simulink model "IndustrialMicrogrid"  (R2023a)
settings: Solver=FixedStepDiscrete  StartTime=0.0  StopTime=10  FixedStep=Ts  RelTol=1e-3
PostLoadFcn:
  | IndustrialMicrogridInputData
  | GfmGridFormingConverterInputParameters
model workspace (MAT data in the model file):
  caseNum = 2
undefined symbols (not defined in the file): base, BESS, DiscIntNeverNeededParam, grid, Grid, gridInverter, machine, microgrid, PV, PVInverter, PVTransformer, scrFactorRg, scrFactorXg, transformer, Ts
libraries: ee_lib x112, eeGeneralControl x104, nesl_utility_internal x64, simulink x56, nesl_utility x37, fl_lib x29, slpidlib x13, eeTransforms x11, eeTotalHarmonicDistorsion x8, eeRmsMeasurement x4, eeSinusoidalMeasurement x4, simulink_extras x2
(part 6 of 14)

== system IndustrialMicrogrid/MG2 Primary Substation/Microgrid Controller 2/Breaker Control  ==
  Bus Element In1 : Inport  PortName=Control Room  Element=ResynchCmd2
  Bus Element In3 : Inport  PortName=Control Room  Element=PlannedIslandCmd2
  Bus Element In6 : Inport  PortName=Control Room  Element=BRKcontrol2
  Bus Element In4 : Inport  PortName=Control Room  Element=BRKcontrol2
  Bus Element In5 : Inport  Port=2  PortName=MGController  Element=IslandMGController2.MGPlannedIsland2.plannedisland
  Bus Element In2 : Inport  Port=2  PortName=MGController  Element=ResynchMGController2.MGResynch2.resynch
  Cast To Double1 : DataTypeConversion  OutDataTypeStr=double  SaturateOnIntegerOverflow=off  RndMeth=Floor
  Logical Operator1 : Logic  Operator=NOT  AllPortsSameDT=off  OutDataTypeStr=boolean
  Logical Operator{2..5} (4 alike) : Logic  AllPortsSameDT=off  OutDataTypeStr=boolean
  Logical Operator6 : Logic  Operator=OR  AllPortsSameDT=off  OutDataTypeStr=boolean
  Logical Operator7 : Logic  Operator=NOT  AllPortsSameDT=off  OutDataTypeStr=boolean
  Breaker : Outport
  wires:
  Logical Operator7/1 -> Logical Operator5/1
  Logical Operator1/1 -> Logical Operator4/1
  Logical Operator5/1 -> Logical Operator6/2
  Logical Operator4/1 -> Logical Operator6/1
  Bus Element In6/1 -> Logical Operator1/1
  Logical Operator6/1 -> Cast To Double1/1
  Bus Element In4/1 -> Logical Operator5/2
  Logical Operator2/1 -> Logical Operator7/1
  Logical Operator3/1 -> Logical Operator4/2
  Bus Element In5/1 -> Logical Operator3/2
  Bus Element In3/1 -> Logical Operator3/1
  Bus Element In1/1 -> Logical Operator2/1
  Bus Element In2/1 -> Logical Operator2/2
  Cast To Double1/1 -> Breaker/1

== system IndustrialMicrogrid/MG2 Primary Substation/Microgrid Controller 2/Frequency Reference ==
  Bus Element In : Inport  PortName=Control Room  Element=ResynchCmd2
  Bus Element In1 : Inport  PortName=Control Room  Element=PowerCmd2
  Bus Element In4 : Inport  PortName=Control Room  Element=BlackStartMG2
  Bus Element In3 : Inport  Port=2  PortName=MGController  Element=BlackStart.Fref2
  Bus Element In2 : Inport  Port=2  PortName=MGController  Element=ResynchMGController2.MGResynch2.synchfrequency
  Constant : Constant  Value=IslandFrequency
  Constant1 : Constant  Value=GridFrequency
  Gain1 : Gain  Gain=1/60
  Sum : Sum  Inputs=|++
  Switch : Switch  Criteria=u2 > Threshold  Threshold=0.5  SaturateOnIntegerOverflow=off  InputSameDT=off
  Switch1 : Switch  Criteria=u2 > Threshold  Threshold=0.5  SaturateOnIntegerOverflow=off  InputSameDT=off
  Switch2 : Switch  Criteria=u2 > Threshold  Threshold=0.5  SaturateOnIntegerOverflow=off  InputSameDT=off
  fref : Outport
  wires:
  Bus Element In4/1 -> Switch1/2
  Constant1/1 -> Switch2/1
  Switch1/1 -> Gain1/1
  Constant/1 -> Sum/2, Switch/3
  Gain1/1 -> fref/1
  Bus Element In2/1 -> Sum/1
  Bus Element In/1 -> Switch/2
  Bus Element In1/1 -> Switch2/2
  Bus Element In3/1 -> Switch1/1
  Switch2/1 -> Switch1/3
  Sum/1 -> Switch/1
  Switch/1 -> Switch2/3

== system IndustrialMicrogrid/MG2 Primary Substation/Microgrid Controller 2/PLL  ==
  In Bus Element : Inport  PortName=mPCC2  Element=Gridvoltage
  In Bus Element1 : Inport  PortName=mPCC2  Element=mPCC2.voltage
  PLL : Subsystem
  PLL start at 0.2 s : Subsystem
  PLL starts at 0.2 s : Subsystem
  PLL1 : Subsystem
  Bus Element Out : Outport  PortName=Grid2  Element=frequency
  Bus Element Out1 : Outport  PortName=Grid2  Element=angle
  Bus Element Out2 : Outport  PortName=Grid2  Element=voltage
  Bus Element Out3 : Outport  Port=2  PortName=Island2  Element=voltage
  Bus Element Out4 : Outport  Port=2  PortName=Island2  Element=frequency
  Bus Element Out5 : Outport  Port=2  PortName=Island2  Element=angle
  wires:
  PLL1/3(mag) -> Bus Element Out3/1
  PLL1/2(angle) -> Bus Element Out5/1
  PLL1/1(fre) -> Bus Element Out4/1
  PLL/3(mag) -> Bus Element Out2/1
  PLL/2(angle) -> Bus Element Out1/1
  PLL/1(fre) -> Bus Element Out/1
  PLL start at 0.2 s/1(Out1) -> PLL/1(abc)
  In Bus Element1/1 -> PLL starts at 0.2 s/1(PCC measurement)
  PLL starts at 0.2 s/1(abc) -> PLL1/1(abc)
  In Bus Element/1 -> PLL start at 0.2 s/1(PCC measurement)

== system IndustrialMicrogrid/MG2 Primary Substation/Microgrid Controller 2/Planned Island ==
  Control Room : Inport
  mPCCPLL 2 : Inport  Port=2
  Bus Creator : BusCreator  Inputs=2
  Control for Zero Powerflow1 : Subsystem  mask(Planned island control parameters){KpPPlannedIsland=microgrid.KpPPlannedIsland2, KiPPlannedIsland=microgrid.KiPPlannedIsland2, KpQPlannedIsland=microgrid.KpQPlannedIsland2, KiQPlannedIsland=microgrid.KiQPlannedIsland2, ZeroActivePowerThreshold=microgrid.zeroActivePowerThreshold2, ZeroReactivePowerThreshold=microgrid.zeroReactivePowerThreshold2, PlannedIslandDelay=microgrid.plannedIslandDelay}
      mask prompts: KpPPlannedIsland "Active Power Planned Island Proportional Gain"; KiPPlannedIsland "Active Power Planned Island Integral Gain"; KpQPlannedIsland "Reactive Power Planned Island Proportional Gain"; KiQPlannedIsland "Reactive Power Planned Island Intergal Gain"; ZeroActivePowerThreshold "Zero Active Power Threshold"; ZeroReactivePowerThreshold "Zero Reactive Power Threshold"; PlannedIslandDelay "Planned Island Delay"
      mask help: Provide planned island control parameters
  IslandMGController2 : Outport
  wires:
  mPCCPLL 2/1 -> Control for Zero Powerflow1/2(mPCCPLL2), Bus Creator/2  "PCC measurments2"
  Control for Zero Powerflow1/1(MGController2) -> Bus Creator/1  "MGPlannedIsland2"
  Bus Creator/1 -> IslandMGController2/1  "IslandMGController2"
  Control Room/1 -> Control for Zero Powerflow1/1(ControlRoom)

== system IndustrialMicrogrid/MG2 Primary Substation/Microgrid Controller 2/Resynchronization ==
  Control Room : Inport
  mPCCPLL : Inport  Port=2
  BESS : Inport  Port=3
  Bus Creator : BusCreator  Inputs=2
  Frequency and voltage matching : Subsystem  mask(Resynchronization control parameters){GridFrequency=grid.frequency, RadToDegree=microgrid.radToDegree, KpFreResynch=microgrid.KpFreResynch2, KiFreResynch=microgrid.KiFreResynch2, KpVolResynch=microgrid.KpVolResynch2, KiVolResynch=microgrid.KiVolResynch2, KpAngResynch=microgrid.KpAngResynch2, KiAngResynch=microgrid.KiAngResynch2, FrequencyThreshold=microgrid.frequencyThreshold, AngleThreshold=microgrid.angleThreshold, VoltageThreshold=microgrid.voltageThreshold, ResynchDelay=microgrid.resynchDelay, kDroop=microgrid.KDroop}
      mask prompts: GridFrequency "Grid Frequency"; RadToDegree "Rad to Degree"; KpFreResynch "Frequency Resynch Proportional Gain"; KiFreResynch "Frequency Resynch Integral Gain"; KpVolResynch "Voltage Resynch Proportional Gain"; KiVolResynch "Voltage Resynch Integral Gain"; KpAngResynch "Angle Resynch Proportional Gain"; KiAngResynch "Angle Resynch Integral Gain"; FrequencyThreshold "Frequency Matching Threshold"; AngleThreshold "Angle Matching Threshold"; VoltageThreshold "Voltage Matching Threshold"; ResynchDelay "Resynch Delay"; kDroop "Voltage Droop"
      mask help: Provide resynchronization control parameters
  ResynchMGController2 : Outport
  wires:
  Control Room/1 -> Frequency and voltage matching/2(ControlRoom)
  Bus Creator/1 -> ResynchMGController2/1  "ResynchMGController2"
  Frequency and voltage matching/1(MGController2) -> Bus Creator/1  "MGResynch2"
  BESS/1 -> Frequency and voltage matching/1(BESS2)
  mPCCPLL/1 -> Bus Creator/2, Frequency and voltage matching/3(mPCCPLL2)  "PCC measurments2"

== system IndustrialMicrogrid/MG2 Primary Substation/Microgrid Controller 2/Voltage Reference ==
  Bus Element In1 : Inport  PortName=Control Room  Element=ResynchCmd2
  Bus Element In2 : Inport  PortName=Control Room  Element=BlackStartMG2
  Bus Element In4 : Inport  Port=2  PortName=MGController  Element=BlackStart.Vref2
  Bus Element In3 : Inport  Port=2  PortName=MGController  Element=ResynchMGController2.MGResynch2.synchvoltagedpr
  Constant9 : Constant  Value=IslandVoltage
  Switch1 : Switch  Criteria=u2 > Threshold  Threshold=0.5  SaturateOnIntegerOverflow=off  InputSameDT=off
  Switch2 : Switch  Criteria=u2 > Threshold  Threshold=0.5  SaturateOnIntegerOverflow=off  InputSameDT=off
  Vref : Outport
  wires:
  Bus Element In3/1 -> Switch1/1
  Constant9/1 -> Switch1/3
  Switch2/1 -> Vref/1
  Bus Element In2/1 -> Switch2/2
  Bus Element In1/1 -> Switch1/2
  Bus Element In4/1 -> Switch2/1
  Switch1/1 -> Switch2/3

== system IndustrialMicrogrid/MG2 Primary Substation/PCC Measurements and PCC Breaker/Grid Current Measurement ==
  Current and Voltage Sensor (Three-Phase)1 : ee_lib/Sensors & Transducers/Current and Voltage Sensor (Three-Phase)  vMeasurementType=ee.enum.vmeasurement.ll  outputUnit=ee.enum.unit.pu  SRated=2.5e6 A*V  VRated=microgrid.voltage V  I_specify=off  I_priority=None  I=[0, 0, 0] A  I_nominal_specify=off  I_nominal_unit=A  I_nominal_value=1  V_specify=off  V_priority=None  V=[0, 0, 0] V  V_nominal_specify=off  V_nominal_unit=V  V_nominal_value=1
      settings: InternalSimscapePortConfiguration="{\"Bottom\":[],\"Left\":[{\"id\":\"N1\",\"label\":\"~1\",\"type\":\"foundation.electrical.three_phase\"}],\"Right\":[{\"id\":\"V_output\",\"label\":\"V\",\"type\":\"output\"},{\"id\":\"I_output\",\"label\":\"I\",\"type\":\"output\"},{\"id\":\"N2\",\"label\":\"~2\",\"type\":\"foundation.electrical.three_phase\"}],\"Top\":[]}"
  PS-Simulink Converter2 : nesl_utility_internal/PS-Simulink Converter  PhysicalDomain=network_engine_domain  SubClassName=ps_output  LeftPortType=input  RightPortType=output  PseudoPeriodic=off  Frequencies=[]  VectorFormat=1-D array  Unit=V  AffineConversion=off
  PS-Simulink Converter3 : nesl_utility_internal/PS-Simulink Converter  PhysicalDomain=network_engine_domain  SubClassName=ps_output  LeftPortType=input  RightPortType=output  PseudoPeriodic=off  Frequencies=[]  VectorFormat=1-D array  Unit=A  AffineConversion=off
  Terminator : Terminator
  ~ : PMIOPort  Side=Left
  "~ " : PMIOPort  Port=2  Side=Right
  "Grid voltage 2 " : Outport
  wires:
  PS-Simulink Converter3/1 -> Terminator/1
  PS-Simulink Converter2/1 -> "Grid voltage 2 "/1
  connections:
  Current and Voltage Sensor (Three-Phase)1/RConn3 -- "~ "/RConn1
  Current and Voltage Sensor (Three-Phase)1/RConn2 -- PS-Simulink Converter3/LConn1
  ~/RConn1 -- Current and Voltage Sensor (Three-Phase)1/LConn1
  Current and Voltage Sensor (Three-Phase)1/RConn1 -- PS-Simulink Converter2/LConn1

== system IndustrialMicrogrid/MG2 Primary Substation/PCC Measurements and PCC Breaker/Grid Power Measurement ==
  Current and Voltage Sensor (Three-Phase) : ee_lib/Sensors & Transducers/Current and Voltage Sensor (Three-Phase)  vMeasurementType=ee.enum.vmeasurement.ll  outputUnit=ee.enum.unit.pu  SRated=2.5e6 A*V  VRated=microgrid.voltage V  I_specify=off  I_priority=None  I=[0, 0, 0] A  I_nominal_specify=off  I_nominal_unit=A  I_nominal_value=1  V_specify=off  V_priority=None  V=[0, 0, 0] V  V_nominal_specify=off  V_nominal_unit=V  V_nominal_value=1
      settings: InternalSimscapePortConfiguration="{\"Bottom\":[],\"Left\":[{\"id\":\"N1\",\"label\":\"~1\",\"type\":\"foundation.electrical.three_phase\"}],\"Right\":[{\"id\":\"V_output\",\"label\":\"V\",\"type\":\"output\"},{\"id\":\"I_output\",\"label\":\"I\",\"type\":\"output\"},{\"id\":\"N2\",\"label\":\"~2\",\"type\":\"foundation.electrical.three_phase\"}],\"Top\":[]}"
  Low-Pass Filter (Discrete or Continuous) : eeGeneralControl/Low-Pass Filter (Discrete or Continuous)  K=1  T=0.1  B=inf  A=-inf  init_option=Inherited from block input  x0=0  Ts=Ts
  Low-Pass Filter (Discrete or Continuous)1 : eeGeneralControl/Low-Pass Filter (Discrete or Continuous)  K=1  T=0.1  B=inf  A=-inf  init_option=Inherited from block input  x0=0  Ts=Ts
  PS-Simulink Converter : nesl_utility_internal/PS-Simulink Converter  PhysicalDomain=network_engine_domain  SubClassName=ps_output  LeftPortType=input  RightPortType=output  PseudoPeriodic=off  Frequencies=[]  VectorFormat=1-D array  Unit=inherit  AffineConversion=off
  PS-Simulink Converter1 : nesl_utility_internal/PS-Simulink Converter  PhysicalDomain=network_engine_domain  SubClassName=ps_output  LeftPortType=input  RightPortType=output  PseudoPeriodic=off  Frequencies=[]  VectorFormat=1-D array  Unit=inherit  AffineConversion=off
  PS-Simulink Converter8 : nesl_utility_internal/PS-Simulink Converter  PhysicalDomain=network_engine_domain  SubClassName=ps_output  LeftPortType=input  RightPortType=output  PseudoPeriodic=off  Frequencies=[]  VectorFormat=1-D array  Unit=MW  AffineConversion=off
  PS-Simulink Converter9 : nesl_utility_internal/PS-Simulink Converter  PhysicalDomain=network_engine_domain  SubClassName=ps_output  LeftPortType=input  RightPortType=output  PseudoPeriodic=off  Frequencies=[]  VectorFormat=1-D array  Unit=MV*A  AffineConversion=off
  Power Sensor (Three-Phase)2 : ee_lib/Sensors & Transducers/Power Sensor (Three-Phase)  load_type=ee.enum.passive.type_balanced.balanced  f0=60 Hz  config=ee.enum.with_neutral.no  rho=1
      settings: InternalSimscapePortConfiguration="{\"Bottom\":[],\"Left\":[{\"id\":\"N1\",\"label\":\"~1\",\"type\":\"foundation.electrical.three_phase\"}],\"Right\":[{\"id\":\"N2\",\"label\":\"~2\",\"type\":\"foundation.electrical.three_phase\"}],\"Top\":[{\"id\":\"Pm\",\"label\":\"P\",\"type\":\"output\"},{\"id\":\"Qm\",\"label\":\"Q\",\"type\":\"output\"}]}"
  ~ : PMIOPort  Side=Left
  "~ " : PMIOPort  Port=2  Side=Right
  Out Bus Element : Outport  PortName=mPCC2  Element=voltage
  Out Bus Element1 : Outport  PortName=mPCC2  Element=current
  Out Bus Element2 : Outport  PortName=mPCC2  Element=activepower
  Out Bus Element3 : Outport  PortName=mPCC2  Element=reactivepower
  wires:
  Low-Pass Filter (Discrete or Continuous)1/1 -> Out Bus Element3/1
  Low-Pass Filter (Discrete or Continuous)/1 -> Out Bus Element2/1
  PS-Simulink Converter1/1 -> Out Bus Element1/1
  PS-Simulink Converter/1 -> Out Bus Element/1
  PS-Simulink Converter9/1 -> Low-Pass Filter (Discrete or Continuous)1/1
  PS-Simulink Converter8/1 -> Low-Pass Filter (Discrete or Continuous)/1
  connections:
  ~/RConn1 -- Power Sensor (Three-Phase)2/LConn1
  PS-Simulink Converter8/LConn1 -- Power Sensor (Three-Phase)2/LConn2
  Current and Voltage Sensor (Three-Phase)/RConn3 -- "~ "/RConn1
  PS-Simulink Converter9/LConn1 -- Power Sensor (Three-Phase)2/LConn3
  Power Sensor (Three-Phase)2/RConn1 -- Current and Voltage Sensor (Three-Phase)/LConn1
  PS-Simulink Converter/LConn1 -- Current and Voltage Sensor (Three-Phase)/RConn1
  Current and Voltage Sensor (Three-Phase)/RConn2 -- PS-Simulink Converter1/LConn1

== system IndustrialMicrogrid/MG2 Processing, Lighting and Auxiliary Loads/Motor Loads/Subsystem ==
  Gain : Gain  Gain=60/(2*pi)
  Ideal Rotational Motion Sensor : fl_lib/Mechanical/Mechanical Sensors/Ideal Rotational Motion Sensor  reference=foundation.enum.MeasurementReference.difference  acceleration_port=false  velocity_port=true  position_port=false  wrap_angle=false  offset=0 rad
      settings: InternalSimscapePortConfiguration="{\"Bottom\":[],\"Left\":[{\"id\":\"R\",\"label\":\"R\",\"type\":\"foundation.mechanical.rotational.rotational\"}],\"Right\":[{\"id\":\"C\",\"label\":\"C\",\"type\":\"foundation.mechanical.rotational.rotational\"},{\"id\":\"W\",\"label\":\"W\",\"type\":\"output\"}],\"Top\":[]}"
  Machine Mechanical Power : ee_lib/Electromechanical/Mechanical/Machine Mechanical Power  power_sign=1  SRated=750000 A*V  FRated=60 Hz  nPolePairs=2  inputUnit=ee.enum.unit.si  torque_factor=2  inertia_option=2  J=10 kg*m^2  H=3.525 W*s/(A*V)  damper_option=2  D=39.0509 N*m*s/rad  pu_D=0.01  initialization_option=1  fMechanical0=30 Hz  fElectrical0=60 Hz
      settings: InternalSimscapePortConfiguration="{\"Bottom\":[],\"Left\":[{\"id\":\"Pm\",\"label\":\"Pm\",\"type\":\"input\"}],\"Right\":[{\"id\":\"R\",\"label\":\"R\",\"type\":\"foundation.mechanical.rotational.rotational\"},{\"id\":\"C\",\"label\":\"C\",\"type\":\"foundation.mechanical.rotational.rotational\"}],\"Top\":[]}"
  Mechanical Rotational Reference : fl_lib/Mechanical/Rotational Elements/Mechanical Rotational Reference
  PS-Simulink Converter : nesl_utility/PS-Simulink Converter  PhysicalDomain=network_engine_domain  SubClassName=ps_output  LeftPortType=input  RightPortType=output  PseudoPeriodic=off  Frequencies=[]  VectorFormat=inherit  Unit=inherit  AffineConversion=off
  Power : Constant  Value=300000  SampleTime=Ts
  Rotational Friction : fl_lib/Mechanical/Rotational Elements/Rotational Friction  brkwy_trq=25 N*m  brkwy_vel=0.1 rad/s  Col_trq=20 N*m  visc_coef=0.001 N*m*s/rad  w_specify=off  w_priority=None  w=0 rad/s  w_nominal_specify=off  w_nominal_unit=rad/s  w_nominal_value=1  t_specify=off  t_priority=None  t=0 N*m  t_nominal_specify=off  t_nominal_unit=N*m  t_nominal_value=1
  Scope : Scope
  Simulink-PS Converter2 : nesl_utility/Simulink-PS Converter  PhysicalDomain=network_engine_domain  SubClassName=ps_input  LeftPortType=input  RightPortType=output  PseudoPeriodic=off  Frequencies=[]  NoiseDistribution=none  NoiseParameters=[]  Unit=1  AffineConversion=off  FilteringAndDerivatives=provide  SimscapeFilterOrder=1  InputFilterTimeConstant=0.001  UdotUserProvided=0
  Conn1 : PMIOPort  Side=Left
  Conn2 : PMIOPort  Port=2  Side=Left
  wires:
  Power/1 -> Simulink-PS Converter2/1
  Gain/1 -> Scope/1
  PS-Simulink Converter/1 -> Gain/1
  connections:
  Ideal Rotational Motion Sensor/RConn1 -- Machine Mechanical Power/RConn2 -- Rotational Friction/RConn1 -- Mechanical Rotational Reference/LConn1 -- Conn2/RConn1
  Machine Mechanical Power/RConn1 -- Rotational Friction/LConn1 -- Ideal Rotational Motion Sensor/LConn1 -- Conn1/RConn1
  Simulink-PS Converter2/RConn1 -- Machine Mechanical Power/LConn1
  PS-Simulink Converter/LConn1 -- Ideal Rotational Motion Sensor/RConn2

== system IndustrialMicrogrid/Operator Room/OperatorControlRoom/MG1 Controller : Commands and Measurements ==
  mLoad : Inport
  MGController1 : Inport  Port=2
  Tieline : Inport  Port=3
  mLoad3 : Inport  Port=4
  "Microgrid Controller 1 : Commands and Measurements" : Subsystem
  Out Bus Element : Outport  PortName=ControlRoom  Element=ResynchCmd
  Out Bus Element1 : Outport  PortName=ControlRoom  Element=PowerCmd
  Out Bus Element2 : Outport  PortName=ControlRoom  Element=Pref
  Out Bus Element3 : Outport  PortName=ControlRoom  Element=Qref
  Out Bus Element4 : Outport  PortName=ControlRoom  Element=Load1Control
  Out Bus Element5 : Outport  PortName=ControlRoom  Element=Load2aControl
  Out Bus Element9 : Outport  PortName=ControlRoom  Element=BRKcontrol
  Out Bus Element6 : Outport  PortName=ControlRoom  Element=PlannedIslandCmd
  Out Bus Element7 : Outport  PortName=ControlRoom  Element=UnitSubstationBrk1
  Out Bus Element8 : Outport  PortName=ControlRoom  Element=UnitSubstationBrk2
  Out Bus Element21 : Outport  PortName=ControlRoom  Element=PortableSubstationBrk1
  Out Bus Element23 : Outport  PortName=ControlRoom  Element=VFMode1
  Out Bus Element31 : Outport  PortName=ControlRoom  Element=BlackStartMG1
  Out Bus Element32 : Outport  PortName=ControlRoom  Element=BlackStartResetMG1
  Out Bus Element33 : Outport  PortName=ControlRoom  Element=Load2bControl
  Out Bus Element34 : Outport  PortName=ControlRoom  Element=Vref1
  Out Bus Element35 : Outport  PortName=ControlRoom  Element=Fref1
  Out Bus Element36 : Outport  PortName=ControlRoom  Element=SubstationBrk
  wires:
  mLoad/1 -> "Microgrid Controller 1 : Commands and Measurements"/1(mLoad)
  MGController1/1 -> "Microgrid Controller 1 : Commands and Measurements"/2(MGController)
  "Microgrid Controller 1 : Commands and Measurements"/18(SubstationBrk) -> Out Bus Element36/1
  "Microgrid Controller 1 : Commands and Measurements"/17(Frequency Setpoint) -> Out Bus Element35/1
  "Microgrid Controller 1 : Commands and Measurements"/11(Portable Substation  BRK1 Control) -> Out Bus Element21/1
  "Microgrid Controller 1 : Commands and Measurements"/10(Unit Substation BRK2 Control) -> Out Bus Element8/1
  "Microgrid Controller 1 : Commands and Measurements"/14(Black Start Reset) -> Out Bus Element32/1
  "Microgrid Controller 1 : Commands and Measurements"/13(Black Start) -> Out Bus Element31/1
  "Microgrid Controller 1 : Commands and Measurements"/9(Unit Substation BRK1 Control) -> Out Bus Element7/1
  "Microgrid Controller 1 : Commands and Measurements"/15(Load 2b Control) -> Out Bus Element33/1
  "Microgrid Controller 1 : Commands and Measurements"/8(Load 2 Control) -> Out Bus Element5/1
  "Microgrid Controller 1 : Commands and Measurements"/7(Load 1 Control) -> Out Bus Element4/1
  "Microgrid Controller 1 : Commands and Measurements"/16(Voltage Setpoint) -> Out Bus Element34/1
  "Microgrid Controller 1 : Commands and Measurements"/1(Resynch_Command) -> Out Bus Element/1
  "Microgrid Controller 1 : Commands and Measurements"/12(VFMode) -> Out Bus Element23/1
  "Microgrid Controller 1 : Commands and Measurements"/3(Power Tracking Command) -> Out Bus Element1/1
  "Microgrid Controller 1 : Commands and Measurements"/2(Planned Island_Command) -> Out Bus Element6/1
  "Microgrid Controller 1 : Commands and Measurements"/5(Active Power setpoint) -> Out Bus Element2/1
  "Microgrid Controller 1 : Commands and Measurements"/6(Reactive Power Setpoint) -> Out Bus Element3/1
  "Microgrid Controller 1 : Commands and Measurements"/4(CB2DisconnectorCommand) -> Out Bus Element9/1
  Tieline/1 -> "Microgrid Controller 1 : Commands and Measurements"/3(Tieline)
  mLoad3/1 -> "Microgrid Controller 1 : Commands and Measurements"/4(mLoad3)

== system IndustrialMicrogrid/Operator Room/OperatorControlRoom/MG2 Controller : Commands and Measurements ==
  mLoad2 : Inport
  MGController2 : Inport  Port=2
  mPV : Inport  Port=3
  mDiesel : Inport  Port=4
  mTieline : Inport  Port=5
  "Microgrid Controller 2 : Commands and Measurements" : Subsystem
  Out Bus Element10 : Outport  PortName=ControlRoom  Element=ResynchCmd2
  Out Bus Element11 : Outport  PortName=ControlRoom  Element=PowerCmd2
  Out Bus Element12 : Outport  PortName=ControlRoom  Element=Pref2
  Out Bus Element13 : Outport  PortName=ControlRoom  Element=Qref2
  Out Bus Element14 : Outport  PortName=ControlRoom  Element=Load3Control
  Out Bus Element15 : Outport  PortName=ControlRoom  Element=Load4aControl
  Out Bus Element16 : Outport  PortName=ControlRoom  Element=BRKcontrol2
  Out Bus Element17 : Outport  PortName=ControlRoom  Element=PlannedIslandCmd2
  Out Bus Element18 : Outport  PortName=ControlRoom  Element=PowerCenterBrk1
  Out Bus Element19 : Outport  PortName=ControlRoom  Element=PowerCenterBrk2
  Out Bus Element20 : Outport  PortName=ControlRoom  Element=PowerCenterDieselBrk
  Out Bus Element22 : Outport  PortName=ControlRoom  Element=Load5Control
  Out Bus Element24 : Outport  PortName=ControlRoom  Element=VFMode2
  Out Bus Element25 : Outport  PortName=ControlRoom  Element=BlackStartMG2
  Out Bus Element26 : Outport  PortName=ControlRoom  Element=Vref2
  Out Bus Element27 : Outport  PortName=ControlRoom  Element=Fref2
  Out Bus Element28 : Outport  PortName=ControlRoom  Element=Load4bControl
  Out Bus Element29 : Outport  PortName=ControlRoom  Element=BlackStartResetMG2
  Out Bus Element37 : Outport  PortName=ControlRoom  Element=PowerCenterBrk3
  Out Bus Element38 : Outport  PortName=ControlRoom  Element=Substation2Brk
  wires:
  mDiesel/1 -> "Microgrid Controller 2 : Commands and Measurements"/4(mdiesel)
  mLoad2/1 -> "Microgrid Controller 2 : Commands and Measurements"/2(mload2)
  mPV/1 -> "Microgrid Controller 2 : Commands and Measurements"/1(mPV)
  MGController2/1 -> "Microgrid Controller 2 : Commands and Measurements"/3(MGController2)
  "Microgrid Controller 2 : Commands and Measurements"/18(BlackStart Reset) -> Out Bus Element29/1
  "Microgrid Controller 2 : Commands and Measurements"/17(Load 4b Control) -> Out Bus Element28/1
  "Microgrid Controller 2 : Commands and Measurements"/15(Voltage setpoint) -> Out Bus Element26/1
  "Microgrid Controller 2 : Commands and Measurements"/16(Frequency setpoint) -> Out Bus Element27/1
  "Microgrid Controller 2 : Commands and Measurements"/14(Black Start) -> Out Bus Element25/1
  "Microgrid Controller 2 : Commands and Measurements"/11(PowerCenter BRK2 Control) -> Out Bus Element19/1
  "Microgrid Controller 2 : Commands and Measurements"/6(Reactive Power Setpoint2) -> Out Bus Element13/1
  "Microgrid Controller 2 : Commands and Measurements"/19(PowerCenter BRK3 Control1) -> Out Bus Element37/1
  "Microgrid Controller 2 : Commands and Measurements"/13(VFMode2) -> Out Bus Element24/1
  "Microgrid Controller 2 : Commands and Measurements"/20(SubstationBrk) -> Out Bus Element38/1
  "Microgrid Controller 2 : Commands and Measurements"/12(PowerCenter Diesel Breaker Control) -> Out Bus Element20/1
  "Microgrid Controller 2 : Commands and Measurements"/9(Load 5 Control) -> Out Bus Element22/1
  "Microgrid Controller 2 : Commands and Measurements"/5(Active Power setpoint2) -> Out Bus Element12/1
  "Microgrid Controller 2 : Commands and Measurements"/4(CB2DisconnectorCommand2) -> Out Bus Element16/1
  "Microgrid Controller 2 : Commands and Measurements"/8(Load 4a Control) -> Out Bus Element15/1
  "Microgrid Controller 2 : Commands and Measurements"/3(Power Tracking Command) -> Out Bus Element11/1
  "Microgrid Controller 2 : Commands and Measurements"/2(Planned Island_Command2) -> Out Bus Element17/1
  "Microgrid Controller 2 : Commands and Measurements"/10(PowerCenterBRK1 Control) -> Out Bus Element18/1
  "Microgrid Controller 2 : Commands and Measurements"/7(Load 3 Control) -> Out Bus Element14/1
  "Microgrid Controller 2 : Commands and Measurements"/1(Resynch_Command2) -> Out Bus Element10/1
  mTieline/1 -> "Microgrid Controller 2 : Commands and Measurements"/5(Tieline)

== system IndustrialMicrogrid/Operator Room/Signal Selector/MG1 Load ==
  In1 : Inport
  Bus Creator4 : BusCreator  Inputs=3
  Bus Selector4 : BusSelector  OutputSignals=Load1Control,Load2aControl,Load2bControl
  Out1 : Outport
  wires:
  Bus Selector4/2 -> Bus Creator4/2  "<Load2aControl>"
  Bus Creator4/1 -> Out1/1
  Bus Selector4/3 -> Bus Creator4/3  "<Load2bControl>"
  Bus Selector4/1 -> Bus Creator4/1  "<Load1Control>"
  In1/1 -> Bus Selector4/1

== system IndustrialMicrogrid/Operator Room/Signal Selector/MG1 Portable Substation ==
  In1 : Inport
  Bus Creator6 : BusCreator  Inputs=1
  Bus Selector6 : BusSelector  OutputSignals=PortableSubstationBrk1
  Portable Substation : Outport
  wires:
  Bus Selector6/1 -> Bus Creator6/1  "<PortableSubstationBrk1>"
  In1/1 -> Bus Selector6/1
  Bus Creator6/1 -> Portable Substation/1

== system IndustrialMicrogrid/Operator Room/Signal Selector/MG1 Primary Substation ==
  In1 : Inport
  Bus Creator : BusCreator  Inputs=12
  Bus Selector : BusSelector  OutputSignals=ResynchCmd,PowerCmd,Pref,Qref,BRKcontrol,PlannedIslandCmd,VFMode1,BlackStartMG1,BlackStartResetMG1,Vref1,Fref1,SubstationBrk
  Primary Substation 1 : Outport
  wires:
  Bus Selector/7 -> Bus Creator/7  "<VFMode1>"
  Bus Selector/11 -> Bus Creator/11  "<Fref1>"
  Bus Selector/10 -> Bus Creator/10  "<Vref1>"
  Bus Selector/3 -> Bus Creator/3  "<Pref>"
  Bus Selector/12 -> Bus Creator/12  "<SubstationBrk>"
  Bus Selector/8 -> Bus Creator/8  "<BlackStartMG1>"
  Bus Selector/4 -> Bus Creator/4  "<Qref>"
  Bus Selector/9 -> Bus Creator/9  "<BlackStartResetMG1>"
  Bus Selector/2 -> Bus Creator/2  "<PowerCmd>"
  Bus Selector/6 -> Bus Creator/6  "<PlannedIslandCmd>"
  Bus Creator/1 -> Primary Substation 1/1
  Bus Selector/5 -> Bus Creator/5  "<BRKcontrol>"
  Bus Selector/1 -> Bus Creator/1  "<ResynchCmd>"
  In1/1 -> Bus Selector/1

== system IndustrialMicrogrid/Operator Room/Signal Selector/MG1 Unit Substation ==
  In1 : Inport
  Bus Creator2 : BusCreator  Inputs=2
  Bus Selector2 : BusSelector  OutputSignals=UnitSubstationBrk1,UnitSubstationBrk2
  Out1 : Outport
  wires:
  Bus Creator2/1 -> Out1/1
  Bus Selector2/2 -> Bus Creator2/2  "<UnitSubstationBrk2>"
  Bus Selector2/1 -> Bus Creator2/1  "<UnitSubstationBrk1>"
  In1/1 -> Bus Selector2/1

== system IndustrialMicrogrid/Operator Room/Signal Selector/MG2 Load ==
  In1 : Inport
  Bus Creator5 : BusCreator  Inputs=4
  Bus Selector5 : BusSelector  OutputSignals=Load3Control,Load4aControl,Load4bControl,Load5Control
  Out1 : Outport
  wires:
  Bus Selector5/2 -> Bus Creator5/2  "<Load4aControl>"
  Bus Selector5/1 -> Bus Creator5/1  "<Load3Control>"
  Bus Selector5/4 -> Bus Creator5/4  "<Load5Control>"
  Bus Selector5/3 -> Bus Creator5/3  "<Load4bControl>"
  In1/1 -> Bus Selector5/1
  Bus Creator5/1 -> Out1/1

== system IndustrialMicrogrid/Operator Room/Signal Selector/MG2 Power Center ==
  In1 : Inport
  Bus Creator3 : BusCreator  Inputs=4
  Bus Selector3 : BusSelector  OutputSignals=PowerCenterBrk1,PowerCenterBrk2,PowerCenterDieselBrk,PowerCenterBrk3
  Out1 : Outport
  wires:
  Bus Selector3/1 -> Bus Creator3/1  "<PowerCenterBrk1>"
  Bus Selector3/2 -> Bus Creator3/2  "<PowerCenterBrk2>"
  Bus Selector3/4 -> Bus Creator3/4  "<PowerCenterBrk3>"
  Bus Selector3/3 -> Bus Creator3/3  "<PowerCenterDieselBrk>"
  In1/1 -> Bus Selector3/1
  Bus Creator3/1 -> Out1/1

== system IndustrialMicrogrid/Operator Room/Signal Selector/MG2 Primary Substation ==
  In1 : Inport
  Bus Creator1 : BusCreator  Inputs=12
  Bus Selector1 : BusSelector  OutputSignals=ResynchCmd2,PowerCmd2,Pref2,Qref2,BRKcontrol2,PlannedIslandCmd2,VFMode2,BlackStartMG2,Vref2,Fref2,BlackStartResetMG2,Substation2Brk
  Primary Substation 2 : Outport
  wires:
  Bus Selector1/5 -> Bus Creator1/5  "<BRKcontrol2>"
  Bus Selector1/3 -> Bus Creator1/3  "<Pref2>"
  Bus Selector1/12 -> Bus Creator1/12  "<Substation2Brk>"
  Bus Selector1/4 -> Bus Creator1/4  "<Qref2>"
  Bus Selector1/2 -> Bus Creator1/2  "<PowerCmd2>"
  Bus Selector1/8 -> Bus Creator1/8  "<BlackStartMG2>"
  Bus Selector1/11 -> Bus Creator1/11  "<BlackStartResetMG2>"
  In1/1 -> Bus Selector1/1
  Bus Selector1/7 -> Bus Creator1/7  "<VFMode2>"
  Bus Selector1/10 -> Bus Creator1/10  "<Fref2>"
  Bus Selector1/1 -> Bus Creator1/1  "<ResynchCmd2>"
  Bus Creator1/1 -> Primary Substation 2/1
  Bus Selector1/9 -> Bus Creator1/9  "<Vref2>"
  Bus Selector1/6 -> Bus Creator1/6  "<PlannedIslandCmd2>"

== system IndustrialMicrogrid/Selected Results/MG1/Inverter Active & Reactive Power  ==
  Vabc : Inport
  Iabc : Inport  Port=2
  Demux : Demux  Outputs=3
  Gain : Gain  Gain=1/sqrt(3)
  Low-Pass Filter (Discrete or Continuous) : eeGeneralControl/Low-Pass Filter (Discrete or Continuous)  K=1  T=0.02  B=inf  A=-inf  init_option=Inherited from block input  x0=0  Ts=-1
  Low-Pass Filter (Discrete or Continuous)1 : eeGeneralControl/Low-Pass Filter (Discrete or Continuous)  K=1  T=0.02  B=inf  A=-inf  init_option=Inherited from block input  x0=0  Ts=-1
  Minus : Sum  Inputs=+-
  Minus1 : Sum  Inputs=+-
  Minus2 : Sum  Inputs=+-
  Mux : Mux  Inputs=3
  Product : Product
  Product1 : Product
  Sum of Elements : Sum  Inputs=+
  Sum of Elements1 : Sum  Inputs=+
  gain : Gain  Gain=2/3
  gain1 : Gain  Gain=2/3
  P : Outport  VectorParamsAs1DForOutWhenUnconnected=off
  Q : Outport  Port=2  VectorParamsAs1DForOutWhenUnconnected=off
  wires:
  Minus/1 -> Mux/3
  Minus2/1 -> Mux/2
  Minus1/1 -> Mux/1
  Gain/1 -> Low-Pass Filter (Discrete or Continuous)1/1
  Sum of Elements1/1 -> Gain/1
  Product1/1 -> Sum of Elements1/1
  Mux/1 -> Product1/2
  Demux/3 -> Minus1/2, Minus2/1
  Demux/2 -> Minus/2, Minus1/1
  Demux/1 -> Minus/1, Minus2/2
  Sum of Elements/1 -> Low-Pass Filter (Discrete or Continuous)/1
  Product/1 -> Sum of Elements/1
  Iabc/1 -> Product/2, Product1/1
  Vabc/1 -> Product/1, Demux/1
  Low-Pass Filter (Discrete or Continuous)/1 -> gain/1
  Low-Pass Filter (Discrete or Continuous)1/1 -> gain1/1
  gain/1 -> P/1  "BESS Active Power(pu)"
  gain1/1 -> Q/1  "BESS Reactive Power(pu)"

== system IndustrialMicrogrid/Selected Results/MG2/Inverter Active & Reactive Power 1 ==
  Vabc : Inport
  Iabc : Inport  Port=2
  Demux : Demux  Outputs=3
  Gain : Gain  Gain=1/sqrt(3)
  Low-Pass Filter (Discrete or Continuous) : eeGeneralControl/Low-Pass Filter (Discrete or Continuous)  K=1  T=0.02  B=inf  A=-inf  init_option=Inherited from block input  x0=0  Ts=-1
  Low-Pass Filter (Discrete or Continuous)1 : eeGeneralControl/Low-Pass Filter (Discrete or Continuous)  K=1  T=0.02  B=inf  A=-inf  init_option=Inherited from block input  x0=0  Ts=-1
  Minus : Sum  Inputs=+-
  Minus1 : Sum  Inputs=+-
  Minus2 : Sum  Inputs=+-
  Mux : Mux  Inputs=3
  Product : Product
  Product1 : Product
  Sum of Elements : Sum  Inputs=+
  Sum of Elements1 : Sum  Inputs=+
  gain : Gain  Gain=2/3
  gain1 : Gain  Gain=2/3
  P : Outport  VectorParamsAs1DForOutWhenUnconnected=off
  Q : Outport  Port=2  VectorParamsAs1DForOutWhenUnconnected=off
  wires:
  gain1/1 -> Q/1  "BESS Reactive Power(pu)"
  gain/1 -> P/1  "BESS Active Power(pu)"
  Low-Pass Filter (Discrete or Continuous)1/1 -> gain1/1
  Low-Pass Filter (Discrete or Continuous)/1 -> gain/1
  Vabc/1 -> Demux/1, Product/1
  Iabc/1 -> Product1/1, Product/2
  Product/1 -> Sum of Elements/1
  Sum of Elements/1 -> Low-Pass Filter (Discrete or Continuous)/1
  Demux/1 -> Minus2/2, Minus/1
  Demux/2 -> Minus1/1, Minus/2
  Demux/3 -> Minus2/1, Minus1/2
  Mux/1 -> Product1/2
  Product1/1 -> Sum of Elements1/1
  Sum of Elements1/1 -> Gain/1
  Gain/1 -> Low-Pass Filter (Discrete or Continuous)1/1
  Minus1/1 -> Mux/1
  Minus2/1 -> Mux/2
  Minus/1 -> Mux/3

== system IndustrialMicrogrid/MG1 Primary Substation/BESS and Controller/BESS/Filter & Sensor ==
  Current Sensor (Three-Phase) : ee_lib/Sensors & Transducers/Current Sensor (Three-Phase)
  Electrical Reference1 : fl_lib/Electrical/Electrical Elements/Electrical Reference
  Low-Pass Filter (Discrete or Continuous)1 : eeGeneralControl/Low-Pass Filter (Discrete or Continuous)  K=1  T=1/(200*gridInverter.frequency)  B=inf  A=-inf  init_option=Specify as parameter  x0=0  Ts=gridInverter.controller.VoltageControlSampleTime
  Low-Pass Filter (Discrete or Continuous)2 : eeGeneralControl/Low-Pass Filter (Discrete or Continuous)  K=1  T=1/(200*gridInverter.frequency)  B=inf  A=-inf  init_option=Specify as parameter  x0=0  Ts=gridInverter.controller.VoltageControlSampleTime
  Neutral Port (Three-Phase) : ee_lib/Connectors & References/Neutral Port (Three-Phase)  G_parasitic=1e-12 1/Ohm
      settings: InternalSimscapePortConfiguration="{\"Bottom\":[],\"Left\":[{\"id\":\"N\",\"label\":\"~\",\"type\":\"foundation.electrical.three_phase\"}],\"Right\":[{\"id\":\"n\",\"label\":\"n\",\"type\":\"foundation.electrical.electrical\"}],\"Top\":[]}"
  PS-Simulink Converter : nesl_utility/PS-Simulink Converter  PhysicalDomain=network_engine_domain  SubClassName=ps_output  LeftPortType=input  RightPortType=output  PseudoPeriodic=off  Frequencies=[]  VectorFormat=inherit  Unit=inherit  AffineConversion=off
  PS-Simulink Converter1 : nesl_utility/PS-Simulink Converter  PhysicalDomain=network_engine_domain  SubClassName=ps_output  LeftPortType=input  RightPortType=output  PseudoPeriodic=off  Frequencies=[]  VectorFormat=inherit  Unit=inherit  AffineConversion=off
  Phase Voltage Sensor (Three-Phase) : ee_lib/Sensors & Transducers/Phase Voltage Sensor (Three-Phase)
  RLC (Three-Phase) : ee_lib/Passive/RLC Assemblies/RLC (Three-Phase)  component_structure=ee.enum.rlc.structure.SeriesRL  R=gridInverter.lineResistance Ohm  L=gridInverter.L*10 H  C=1e-6 F  R_parasitic=0 Ohm  G_parasitic=0 1/Ohm  IL_specify=off  IL_priority=High  IL=[0, 0, 0] A  IL_nominal_specify=off  IL_nominal_unit=A  IL_nominal_value=1  VC_specify=off  VC_priority=High  VC=[0, 0, 0] V  VC_nominal_specify=off  VC_nominal_unit=V  VC_nominal_value=1
      settings: InternalSimscapePortConfiguration="{\"Bottom\":[],\"Left\":[{\"id\":\"N1\",\"label\":\"~1\",\"type\":\"foundation.electrical.three_phase\"}],\"Right\":[{\"id\":\"N2\",\"label\":\"~2\",\"type\":\"foundation.electrical.three_phase\"}],\"Top\":[]}"
  Inabc : PMIOPort  Side=Left
  Opabc : PMIOPort  Port=2  Side=Right
  Iabc : Outport
  Vabc : Outport  Port=2
  wires:
  PS-Simulink Converter1/1 -> Low-Pass Filter (Discrete or Continuous)1/1
  Low-Pass Filter (Discrete or Continuous)2/1 -> Iabc/1
  PS-Simulink Converter/1 -> Low-Pass Filter (Discrete or Continuous)2/1
  Low-Pass Filter (Discrete or Continuous)1/1 -> Vabc/1
  connections:
  Electrical Reference1/LConn1 -- Neutral Port (Three-Phase)/RConn1
  PS-Simulink Converter1/LConn1 -- Phase Voltage Sensor (Three-Phase)/RConn1
  Current Sensor (Three-Phase)/RConn2 -- RLC (Three-Phase)/LConn1
  Neutral Port (Three-Phase)/LConn1 -- Phase Voltage Sensor (Three-Phase)/RConn2
  Current Sensor (Three-Phase)/LConn1 -- Inabc/RConn1
  PS-Simulink Converter/LConn1 -- Current Sensor (Three-Phase)/RConn1
  Phase Voltage Sensor (Three-Phase)/LConn1 -- Opabc/RConn1 -- RLC (Three-Phase)/RConn1

== system IndustrialMicrogrid/MG1 Primary Substation/BESS and Controller/BESS/Grid-Forming Converter Control ==
  Pref : Inport
  Qref : Inport  Port=2
  Vref : Inport  Port=3
  Fref : Inport  Port=4
  CntrlFlag : Inport  Port=5
  Igabc : Inport  Port=6
  Vgabc : Inport  Port=7
  BlackStart : Inport  Port=8
  Current Limiting : Subsystem
  Grid Voltage Reactive Power Support : Subsystem
  Measurement : Subsystem
      mask Display: image('$imagefile'); % Use "Edit Image" on toolstrip to change.
  Power Control : Subsystem
  VoltageCurrentControl : Subsystem
  mabc : Outport
  Pmeas : Outport  Port=2
  Qmeas : Outport  Port=3
  fmeas : Outport  Port=4
  wires:
  VoltageCurrentControl/1(mabc) -> mabc/1
  Vgabc/1 -> Measurement/1(Vgabcc)
  Igabc/1 -> Measurement/2(Igabc)
  Measurement/2(Pmeas) -> Pmeas/1
  Measurement/3(Qmeas) -> Qmeas/1
  Measurement/1(measure) -> Current Limiting/1(measure), VoltageCurrentControl/1(measure), Power Control/1(measure), Grid Voltage Reactive Power Support/1(measure)
  Power Control/3(angle) -> Measurement/3(Angle)
  Power Control/1(reactiveControl) -> Current Limiting/2(reactiveControl)
  Power Control/2(activeControl) -> VoltageCurrentControl/3(activeControl)
  Current Limiting/1(currentLimiting) -> VoltageCurrentControl/2(currentLimiting)
  Qref/1 -> Grid Voltage Reactive Power Support/3(QrefInput)
  Pref/1 -> Grid Voltage Reactive Power Support/2(PrefInput)
  Grid Voltage Reactive Power Support/1(Pref) -> Power Control/2(Pref)
  Grid Voltage Reactive Power Support/2(Qref) -> Power Control/3(Qref)
  Measurement/4(fmeas) -> fmeas/1
  Fref/1 -> Power Control/5(Fref)
  Vref/1 -> Power Control/4(Vref)
  CntrlFlag/1 -> Power Control/6(CntrlFlag)
  BlackStart/1 -> VoltageCurrentControl/4(BlackStart)

== system IndustrialMicrogrid/MG1 Primary Substation/BESS and Controller/BESS/Per Unit Conversion ==
  fgrid : Inport
  Vabc : Inport  Port=2
  Iabc : Inport  Port=3
  Amp2PU : Gain  Gain=1/base.current
  PU2Hz : Gain  Gain=gridInverter.frequency
  Volt2PU : Gain  Gain=1/base.voltage
  fmeasHz : Outport
  Vabcpu : Outport  Port=2
  Iabcpu : Outport  Port=3
  wires:
  PU2Hz/1 -> fmeasHz/1
  fgrid/1 -> PU2Hz/1
  Volt2PU/1 -> Vabcpu/1  "Vabc"
  Iabc/1 -> Amp2PU/1
  Amp2PU/1 -> Iabcpu/1  "Iabc"
  Vabc/1 -> Volt2PU/1

== system IndustrialMicrogrid/MG1 Primary Substation/BESS and Controller/BESS/Subsystem ==
  PQref : Inport
  Demux : Demux  Outputs=2
  Low-Pass Filter (Discrete or Continuous) : eeGeneralControl/Low-Pass Filter (Discrete or Continuous)  K=1  T=5e-2  B=inf  A=-inf  init_option=Inherited from block input  x0=0  Ts=-1
  Low-Pass Filter (Discrete or Continuous)1 : eeGeneralControl/Low-Pass Filter (Discrete or Continuous)  K=1  T=5e-2  B=inf  A=-inf  init_option=Inherited from block input  x0=0  Ts=-1
  Unit Delay : UnitDelay  SampleTime=-1  HasFrameUpgradeWarning=on
  Unit Delay1 : UnitDelay  SampleTime=-1  HasFrameUpgradeWarning=on
  Pref : Outport
  Qref : Outport  Port=2
  wires:
  Demux/1 -> Unit Delay/1
  Demux/2 -> Unit Delay1/1  "Qref"
  Low-Pass Filter (Discrete or Continuous)/1 -> Pref/1
  Low-Pass Filter (Discrete or Continuous)1/1 -> Qref/1
  PQref/1 -> Demux/1
  Unit Delay/1 -> Low-Pass Filter (Discrete or Continuous)/1
  Unit Delay1/1 -> Low-Pass Filter (Discrete or Continuous)1/1

== system IndustrialMicrogrid/MG1 Primary Substation/BESS and Controller/BESS/Subsystem2 ==
  In1 : Inport
  In2 : Inport  Port=2
  AND : Logic  IconShape=distinctive  AllPortsSameDT=off  OutDataTypeStr=boolean
  Constant : Constant  Value=0
  Delay : Delay  DelayLength=microgrid.controller1BlackStartDelay  SampleTime=Ts*5000
  NOT : Logic  Operator=NOT  IconShape=distinctive  AllPortsSameDT=off  OutDataTypeStr=boolean
  Simulink-PS Converter : nesl_utility/Simulink-PS Converter  PhysicalDomain=network_engine_domain  SubClassName=ps_input  LeftPortType=input  RightPortType=output  PseudoPeriodic=off  Frequencies=[]  NoiseDistribution=none  NoiseParameters=[]  Unit=1  AffineConversion=off  FilteringAndDerivatives=provide  SimscapeFilterOrder=1  InputFilterTimeConstant=0.001  UdotUserProvided=0
  Switch : Switch  Criteria=u2 > Threshold  Threshold=0.5  SaturateOnIntegerOverflow=off  InputSameDT=off
  output : PMIOPort  Side=Right
  wires:
  AND/1 -> Switch/2
  Switch/1 -> Simulink-PS Converter/1
  In2/1 -> Switch/3
  In1/1 -> AND/1, Delay/1
  NOT/1 -> AND/2
  Constant/1 -> Switch/1
  Delay/1 -> NOT/1
  connections:
  Simulink-PS Converter/RConn1 -- output/RConn1

== system IndustrialMicrogrid/MG1 Primary Substation/BESS and Controller/BESS output filter and transformer/Transformer 1 kV//13.8 kV ==
  "Transformer " : ee_lib/Passive/Transformers/Two-Winding Transformer (Three-Phase)  SRated=base.power*1e3 A*V  FRated=gridInverter.frequency Hz  Winding1Connection=ee.enum.windingconnection.Yg  VRated1=transformer.primaryRMSVoltage V  Winding2Connection=ee.enum.windingconnection.delta1  VRated2=transformer.secondaryRMSVoltage V  CoreType=ee.enum.coretype.threelimb  pu_Rw1=transformer.PrimaryResistancePU%*scrFactorRg  pu_Rw2=transformer.SecondaryResistancePU%*scrFactorRg  leakage_reactance_option=ee.enum.transformer_leakage.include  pu_Xl1=transformer.PrimaryReactancePU%*scrFactorXg  pu_Xl2=transformer.SecondaryReactancePU%*scrFactorXg  magnetizing_resistance_option=ee.enum.transformer_magnetizingResistance.exclude  pu_Rm=500  magnetizing_reactance_option=ee.enum.transformer_magnetizingReactance.exclude  saturation_option=ee.enum.transformer_saturation.exclude  pu_Xm=500  current_data=[0, .002, 1, 2]  magnetic_flux_data=[0, 1.2, 1.5, 1.51]  pu_X0=transformer.ZeroSequenceReactancePU%*scrFactorXg*1.1  i1_specify=on  i1_priority=None  i1=[0, 0, 0] A  i1_nominal_specify=off  i1_nominal_unit=A  i1_nominal_value=1  i2_specify=on  i2_priority=None  i2=[0, 0, 0] A  i2_nominal_specify=off  i2_nominal_unit=A  i2_nominal_value=1  phi_specify=off  phi_priority=None  phi=[0, 0, 0]  phi_nominal_specify=off  phi_nominal_unit=1  phi_nominal_value=1  power_dissipated_specify=off  power_dissipated_priority=None  power_dissipated=0 W  power_dissipated_nominal_specify=off  power_dissipated_nominal_unit=W  power_dissipated_nominal_value=1
      settings: InternalSimscapePortConfiguration="{\"Bottom\":[],\"Left\":[{\"id\":\"N1\",\"label\":\"~1\",\"type\":\"foundation.electrical.three_phase\"}],\"Right\":[{\"id\":\"N2\",\"label\":\"~2\",\"type\":\"foundation.electrical.three_phase\"}],\"Top\":[]}"
  ABC1 : PMIOPort  Side=Left
  ABC2 : PMIOPort  Port=2  Side=Right
  connections:
  "Transformer "/RConn1 -- ABC2/RConn1
  "Transformer "/LConn1 -- ABC1/RConn1

== system IndustrialMicrogrid/MG1 Primary Substation/Microgrid Controller/Black Start/If Action Subsystem ==
  Action Port : ActionPort  ActionPortLabel=if(u1 > 0)
  Constant : Constant  Value=60
  Subsystem : Subsystem
  Subsystem1 : Subsystem
  Subsystem2 : Subsystem
  Sum : Sum  Inputs=+++
  Out1 : Outport
  Out2 : Outport  Port=2
  wires:
  Constant/1 -> Out2/1
  Sum/1 -> Out1/1
  Subsystem2/1(Out1) -> Sum/1
  Subsystem/1(Out1) -> Sum/3
  Subsystem1/1(Out1) -> Sum/2

== system IndustrialMicrogrid/MG1 Primary Substation/Microgrid Controller/Black Start/If Action Subsystem1 ==
  Control Room : Inport
  Control Room1 : Inport  Port=2
  Action Port : ActionPort  ActionPortLabel=else
  Out1 : Outport
  Out2 : Outport  Port=2
  wires:
  Control Room/1 -> Out1/1
  Control Room1/1 -> Out2/1

== system IndustrialMicrogrid/MG1 Primary Substation/Microgrid Controller/PLL/PLL ==
  abc : Inport
  Rate Transition : RateTransition  Commented=through
  "Sinusoidal Measurement (PLL, Three-Phase)" : eeSinusoidalMeasurement/Sinusoidal Measurement (PLL, Three-Phase)  Kp_LF=KpPLLController1  Ki_LF=KiPLLController1  F0=GridFrequency  Theta0=0  Ts=Ts
  Subsystem : Subsystem
  fre : Outport
  angle : Outport  Port=2
  mag : Outport  Port=3
  wires:
  abc/1 -> "Sinusoidal Measurement (PLL, Three-Phase)"/1
  "Sinusoidal Measurement (PLL, Three-Phase)"/3 -> Rate Transition/1
  Rate Transition/1 -> mag/1
  "Sinusoidal Measurement (PLL, Three-Phase)"/2 -> Subsystem/1(In)
  Subsystem/1(Out) -> angle/1
  "Sinusoidal Measurement (PLL, Three-Phase)"/1 -> fre/1

== system IndustrialMicrogrid/MG1 Primary Substation/Microgrid Controller/PLL/PLL start at 0.2 s ==
  PCC measurement : Inport
  Constant : Constant  Value=0
  Step : Step  Time=0.2  SampleTime=Ts
  Switch : Switch  Criteria=u2 > Threshold  Threshold=0.5  SaturateOnIntegerOverflow=off  InputSameDT=off
  Out1 : Outport
  wires:
  PCC measurement/1 -> Switch/1
  Switch/1 -> Out1/1
  Constant/1 -> Switch/3
  Step/1 -> Switch/2

== system IndustrialMicrogrid/MG1 Primary Substation/Microgrid Controller/PLL/PLL starts at 0.2 s ==
  PCC measurement : Inport
  Constant1 : Constant  Value=0
  Step : Step  Time=0.2  SampleTime=Ts
  Switch : Switch  Criteria=u2 > Threshold  Threshold=0.5  SaturateOnIntegerOverflow=off  InputSameDT=off
  abc : Outport
  wires:
  PCC measurement/1 -> Switch/1
  Constant1/1 -> Switch/3
  Switch/1 -> abc/1
  Step/1 -> Switch/2

== system IndustrialMicrogrid/MG1 Primary Substation/Microgrid Controller/PLL/PLL1 ==
  abc : Inport
  "Sinusoidal Measurement (PLL, Three-Phase)" : eeSinusoidalMeasurement/Sinusoidal Measurement (PLL, Three-Phase)  Kp_LF=KpPLLController1  Ki_LF=KiPLLController1  F0=GridFrequency  Theta0=0  Ts=Ts
  Subsystem : Subsystem
  fre : Outport
  angle : Outport  Port=2
  mag : Outport  Port=3
  wires:
  "Sinusoidal Measurement (PLL, Three-Phase)"/1 -> fre/1
  Subsystem/1(Out) -> angle/1
  "Sinusoidal Measurement (PLL, Three-Phase)"/2 -> Subsystem/1(In)
  "Sinusoidal Measurement (PLL, Three-Phase)"/3 -> mag/1
  abc/1 -> "Sinusoidal Measurement (PLL, Three-Phase)"/1
